simulink model "Design2_1"  (R2024a)
settings: Solver=VariableStepAuto  StartTime=0.0  StopTime=180  RelTol=1e-3
settings Model: Creator=ALCOT161  LastModifiedBy=ALCOT161

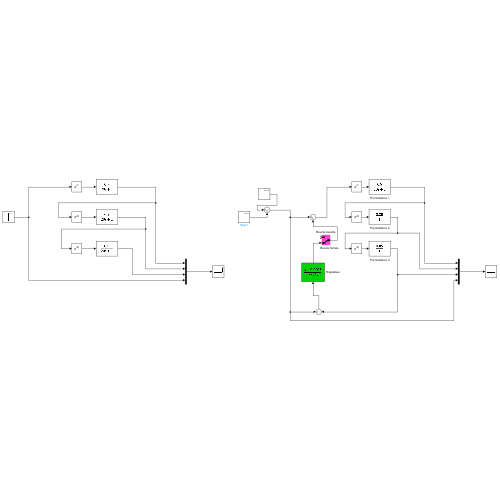
[thumbnail: Simulink's stored preview of the top-level diagram]
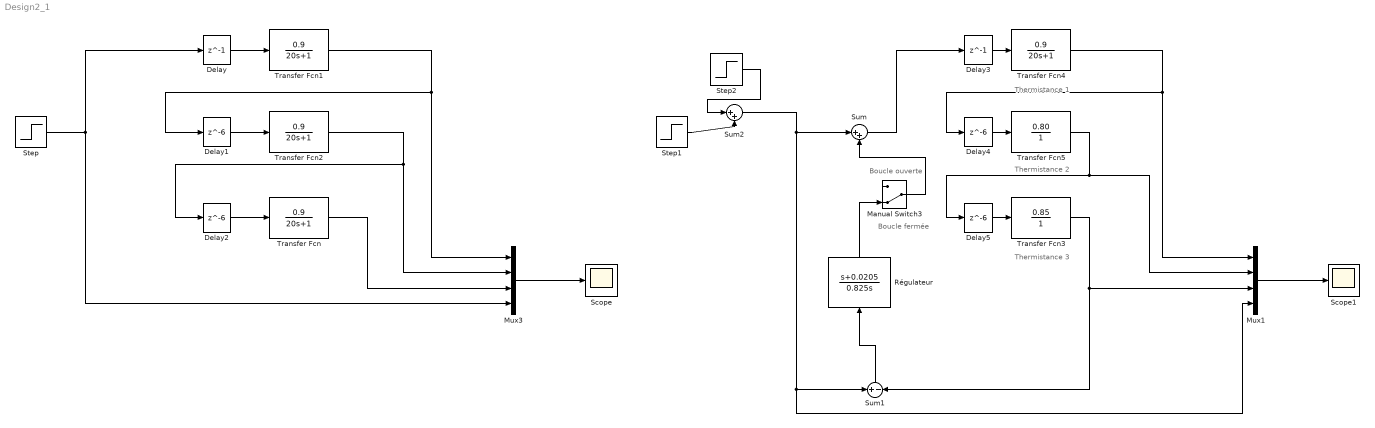
== system Design2_1 ==
  note: Thermistance 3
  note: Thermistance 2
  note: Thermistance 1
  note: Boucle fermée
  note: Boucle ouverte
  Delay : Delay  DelayLength=1  InitialCondition=0  SampleTime=1
  Delay{1..2,4..5} (4 alike) : Delay  DelayLength=6  InitialCondition=0  SampleTime=1
  Delay3 : Delay  DelayLength=1  InitialCondition=0  SampleTime=1
  Manual Switch3 : ManualSwitch  CurrentSetting=0
  Mux1 : Mux
  Mux3 : Mux
  Régulateur : TransferFcn  Numerator=[1 0.0205]  Denominator=[0.825 0]
  Scope : Scope
  Scope1 : Scope
  Step : Step  Time=0  After=25  SampleTime=180
  Step1 : Step  Time=0  After=25  SampleTime=180
  Step2 : Step  Time=10  SampleTime=100
  Sum : Sum  Inputs=|++
  Sum1 : Sum  Inputs=+|-  SampleTime=0
  Sum2 : Sum  Inputs=|++
  Transfer Fcn{,1..2,4} (4 alike) : TransferFcn  Numerator=[0.9]  Denominator=[20 1]
  Transfer Fcn3 : TransferFcn  Numerator=[0.85]  Denominator=[1]
  Transfer Fcn5 : TransferFcn  Numerator=[0.80]  Denominator=[1]
  wires:
  Mux3/1 -> Scope/1
  Delay/1 -> Transfer Fcn1/1
  Delay1/1 -> Transfer Fcn2/1
  Delay2/1 -> Transfer Fcn/1
  Step/1 -> Mux3/4, Delay/1
  Transfer Fcn1/1 -> Delay1/1, Mux3/1
  Transfer Fcn2/1 -> Mux3/2, Delay2/1
  Transfer Fcn/1 -> Mux3/3
  Delay5/1 -> Transfer Fcn3/1
  Transfer Fcn5/1 -> Mux1/2, Delay5/1
  Delay3/1 -> Transfer Fcn4/1
  Delay4/1 -> Transfer Fcn5/1
  Mux1/1 -> Scope1/1
  Transfer Fcn4/1 -> Delay4/1, Mux1/1
  Transfer Fcn3/1 -> Mux1/3, Sum1/2
  Sum1/1 -> Régulateur/1
  Sum/1 -> Delay3/1
  Manual Switch3/1 -> Sum/2
  Régulateur/1 -> Manual Switch3/2
  Step2/1 -> Sum2/1
  Sum2/1 -> Sum1/1, Mux1/4, Sum/1
  Step1/1 -> Sum2/2
